simulink model "test_beam_model"  (R2020b)
settings: Solver=ode15s  StartTime=0.0  StopTime=10  RelTol=1e-3
undefined symbols (not defined in the file): const, mech
settings Model: Creator=Utente  LastModifiedBy=Utente

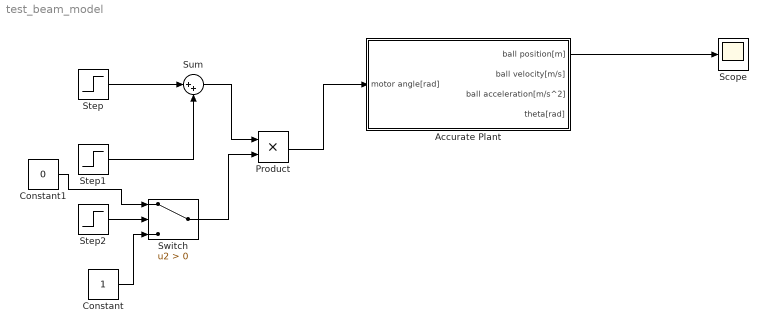
== system test_beam_model ==
  Accurate Plant : Subsystem
  Constant : Constant
  Constant1 : Constant  Value=0
  Product : Product
  Scope : Scope
  Step : Step  Time=0  After=-pi/6  SampleTime=0
  Step1 : Step  After=pi/3  SampleTime=0
  Step2 : Step  Time=2  SampleTime=0
  Sum : Sum  Inputs=|++
  Switch : Switch  Criteria=u2 > Threshold
  wires:
  Accurate Plant/1(ball position[m]) -> Scope/1
  Step/1 -> Sum/1
  Step1/1 -> Sum/2
  Sum/1 -> Product/1
  Step2/1 -> Switch/2
  Switch/1 -> Product/2
  Product/1 -> Accurate Plant/1(motor angle[rad])
  Constant/1 -> Switch/3
  Constant1/1 -> Switch/1

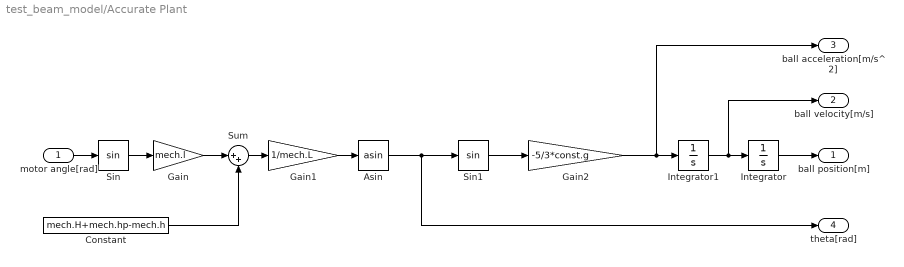
== system test_beam_model/Accurate Plant ==
  motor angle[rad] : Inport
  Asin : Trigonometry  Operator=asin
  Constant : Constant  Value=mech.H+mech.hp-mech.h
  Gain : Gain  Gain=mech.l
  Gain1 : Gain  Gain=1/mech.L
  Gain2 : Gain  Gain=-5/3*const.g
  Integrator : Integrator
  Integrator1 : Integrator
  Sin : Trigonometry
  Sin1 : Trigonometry
  Sum : Sum  Inputs=|++
  ball position[m] : Outport
  ball velocity[m/s] : Outport  Port=2
  ball acceleration[m/s^2] : Outport  Port=3
  theta[rad] : Outport  Port=4
  wires:
  Integrator/1 -> ball position[m]/1
  Integrator1/1 -> ball velocity[m/s]/1, Integrator/1
  Gain2/1 -> ball acceleration[m/s^2]/1, Integrator1/1
  motor angle[rad]/1 -> Sin/1
  Sin/1 -> Gain/1
  Gain/1 -> Sum/1
  Constant/1 -> Sum/2
  Sum/1 -> Gain1/1
  Gain1/1 -> Asin/1
  Sin1/1 -> Gain2/1
  Asin/1 -> theta[rad]/1, Sin1/1
